simulink model "flightSimulation"  (R2018a)
settings: Solver=FixedStepAuto  StartTime=0  StopTime=end_time  FixedStep=0.005  RelTol=1e-3  EnableMultiTasking=on
values from neighbouring files (symbols this model uses):
  initPosLLA = [37.6287386167 -122.393391133 100]    [cmdh.mat]    (also in cmdyaw.mat)
  mass = 1.53    [cmdh.mat]    (also in cmdyaw.mat)
  Ts = 0.01    [cmdh.mat]    (also in cmdyaw.mat)
undefined symbols (not defined in the file or in its folder): B, Earth, ft, m, p_limits, s, sigbuilder_block, sw_turb, umax, umin, Vehicle, WGS84
libraries: simulink x23, aerolibactuator x15, dspswit3 x12, dspsrcs4 x10, dsparch4 x7, aerolibconvert2 x4, aerolibanimutils x2, qcatlib x2, aerolibfltsims x2, aerolibutil x2, shared6dof x1, aerolibtransform2 x1
(part 3 of 4)

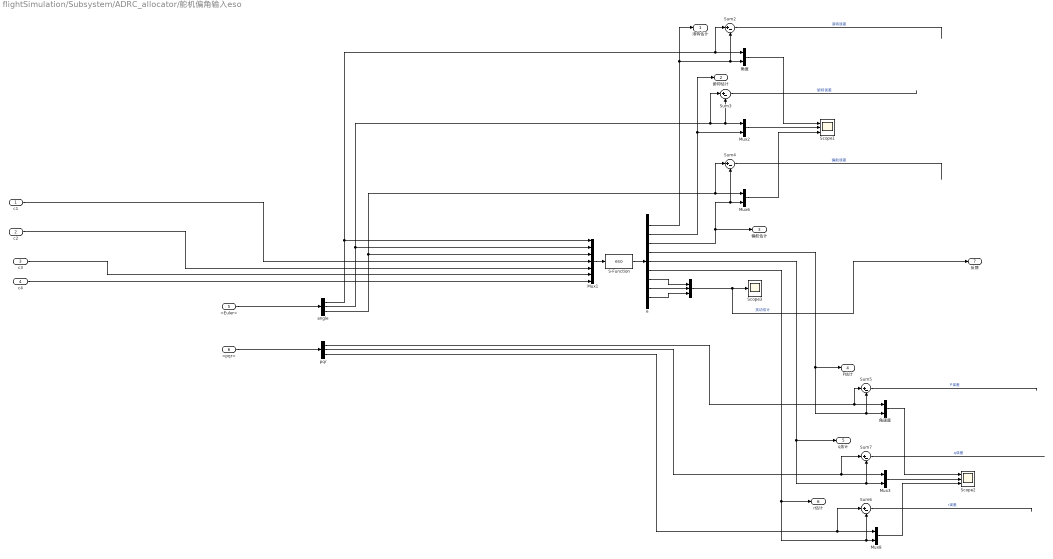
== system flightSimulation/Subsystem/ADRC_allocator/舵机偏角输入eso ==
  c1 : Inport
  c2 : Inport  Port=2
  c3 : Inport  Port=3
  c4 : Inport  Port=4
  <Euler> : Inport  Port=5
  <pqr> : Inport  Port=6
  " " : Mux  Inputs=3
  Mux1 : Mux  Inputs=7
  Mux{2..3,6,8} (4 alike) : Mux  Inputs=2
  S-Function : S-Function  FunctionName=eso  SFunctionDeploymentMode=off  EnableBusSupport=off
  Scope1 : Scope  NumInputPorts=3
  Scope2 : Scope  NumInputPorts=3
  Scope3 : Scope
  Sum{2..7} (6 alike) : Sum  Inputs=|+-
  angle : Demux  Outputs=3
  e : Demux  Outputs=9
  pqr : Demux  Outputs=3
  角度 : Mux  Inputs=2
  角速度 : Mux  Inputs=2
  滚转估计 : Outport
  俯仰估计 : Outport  Port=2
  偏航估计 : Outport  Port=3
  P估计 : Outport  Port=4
  q估计 : Outport  Port=5
  r估计 : Outport  Port=6
  反馈 : Outport  Port=7
  wires:
  e/1 -> 滚转估计/1, Sum2/2, 角度/2
  e/4 -> P估计/1, Sum5/2, 角速度/2
  pqr/1 -> Sum5/1, 角速度/1
  angle/1 -> Sum2/1, 角度/1, Mux1/1
  c3/1 -> Mux1/6
  Sum4/1 -> ?  "偏航误差"
  e/8 -> " "/2
  angle/2 -> Mux2/1, Sum3/2, Sum3/1, Mux1/2
  c2/1 -> Mux1/5
  e/6 -> r估计/1, Mux8/2, Sum6/2
  e/5 -> q估计/1, Sum7/2, Mux3/2
  c4/1 -> Mux1/7
  angle/3 -> Sum4/1, Mux6/1, Mux1/3
  角速度/1 -> Scope2/1
  Mux3/1 -> Scope2/2
  e/3 -> 偏航估计/1, Sum4/2, Mux6/2
  Sum5/1 -> ?  "P误差"
  pqr/3 -> Sum6/1, Mux8/1
  角度/1 -> Scope1/1
  S-Function/1 -> e/1
  pqr/2 -> Sum7/1, Mux3/1
  <Euler>/1 -> angle/1
  Mux6/1 -> Scope1/3
  e/2 -> 俯仰估计/1, Mux2/2
  Mux2/1 -> Scope1/2
  e/7 -> " "/1
  Sum7/1 -> ?  "q误差"
  Mux1/1 -> S-Function/1
  Mux8/1 -> Scope2/3
  e/9 -> " "/3
  Sum6/1 -> ?  "r误差"
  c1/1 -> Mux1/4
  Sum3/1 -> ?  "俯仰误差"
  Sum2/1 -> ?  "滚转误差"
  <pqr>/1 -> pqr/1
  " "/1 -> 反馈/1, Scope3/1  "扰动估计"

== system flightSimulation/Subsystem/ADRC_allocator1/Subsystem ==
  q : Inport
  p : Inport  Port=2
  In3 : Inport  Port=3
  Divide : Product  Inputs=*/
  Gain : Gain  Gain=-1225^2/9.788
  Product : Product
  Saturation1 : Saturate  UpperLimit=1  LowerLimit=0.5
  Sqrt : Sqrt  SaturateOnIntegerOverflow=on
  Trigonometric Function : Trigonometry  Operator=cos
  Trigonometric Function1 : Trigonometry  Operator=cos
  speed : Outport
  wires:
  Saturation1/1 -> Divide/2
  Trigonometric Function/1 -> Product/1
  In3/1 -> Divide/1
  Trigonometric Function1/1 -> Product/2
  p/1 -> Trigonometric Function/1
  Product/1 -> Saturation1/1
  q/1 -> Trigonometric Function1/1
  Divide/1 -> Gain/1
  Gain/1 -> Sqrt/1
  Sqrt/1 -> speed/1

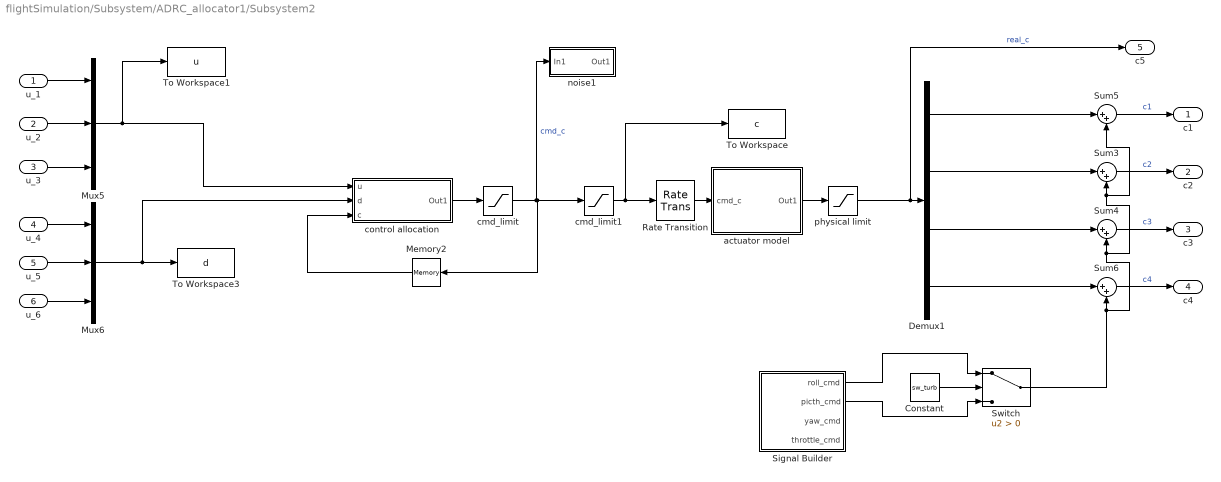
== system flightSimulation/Subsystem/ADRC_allocator1/Subsystem2 ==
  u_1 : Inport
  u_2 : Inport  Port=2
  u_3 : Inport  Port=3
  u_4 : Inport  Port=4
  u_5 : Inport  Port=5
  u_6 : Inport  Port=6
  Constant : Constant  Value=sw_turb
  Demux1 : Demux
  Memory2 : Memory  InitialCondition=[0;0;0;0]  InheritSampleTime=on  LinearizeAsDelay=on
  Mux5 : Mux  Inputs=3
  Mux6 : Mux  Inputs=3
  Rate Transition : RateTransition
  Signal Builder : Subsystem  Tag=STV Subsys  LoadFcn=sigbuilder_block('load');  StartFcn=sigbuilder_block('start');  StopFcn=sigbuilder_block('stop');  ClipboardFcn=sigbuilder_block('clipboard');  mask(Sigbuilder block){tuvar=[0:10]}
      mask help: Simulink:masks:SigbuilderBlock_MD
      mask init:
      | if ~strcmp(get_param(bdroot(gcbh),'SimulationStatus'),'stopped') tuvar = sigbuilder_block('maskInit'); end
      settings: CopyFcn=sigbuilder_block('copy');  DeleteFcn=sigbuilder_block('delete');  ModelCloseFcn=sigbuilder_block('modelClose');  PreSaveFcn=sigbuilder_block('preSave');  PauseFcn=sigbuilder_block('pause');  ContinueFcn=sigbuilder_block('continue');  NameChangeFcn=sigbuilder_block('namechange');  OpenFcn=sigbuilder_block('open',[336 114 630 307.5 ]);  CloseFcn=sigbuilder_block('close');
      mask Display: plot(0, 0, 100, 100,[2, 2, 32, 32, 2], [68, 8, 8, 68, 68],[32, 2], [38, 38], [32, 19, 2],[53, 60, 44], [32, 17, 17, 2],[16, 16, 31, 31]);txt = getActiveGroup(gcbh);text(2, 100, txt,'verticalAlignment', 'top');
  Sum{3..6} (4 alike) : Sum  Inputs=|++
  Switch : Switch  Criteria=u2 > Threshold
  To Workspace : ToWorkspace  VariableName=c  SaveFormat=Timeseries  SampleTime=0.01
  To Workspace1 : ToWorkspace  VariableName=u  SaveFormat=Timeseries  SampleTime=0.01
  To Workspace3 : ToWorkspace  VariableName=d  SaveFormat=Timeseries  SampleTime=0.01
  actuator model : Subsystem
  cmd_limit : Saturate  UpperLimit=umax  LowerLimit=umin
  cmd_limit1 : Saturate  UpperLimit=umax  LowerLimit=umin
  control allocation : Subsystem  Variant=on
  noise1 : Subsystem
  physical limit : Saturate  UpperLimit=umax  LowerLimit=umin
  c1 : Outport
  c2 : Outport  Port=2
  c3 : Outport  Port=3
  c4 : Outport  Port=4
  c5 : Outport  Port=5
  wires:
  u_3/1 -> Mux5/3
  u_1/1 -> Mux5/1
  u_2/1 -> Mux5/2
  u_4/1 -> Mux6/1
  u_5/1 -> Mux6/2
  u_6/1 -> Mux6/3
  Sum5/1 -> c1/1  "c1"
  Sum3/1 -> c2/1  "c2"
  Sum4/1 -> c3/1  "c3"
  Sum6/1 -> c4/1  "c4"
  Memory2/1 -> control allocation/3(c)
  Demux1/1 -> Sum5/1
  Demux1/2 -> Sum3/1
  Demux1/3 -> Sum4/1
  Demux1/4 -> Sum6/1
  Mux6/1 -> control allocation/2(d), To Workspace3/1
  control allocation/1(Out1) -> cmd_limit/1
  Signal Builder/1(roll_cmd) -> Switch/1
  Signal Builder/2(picth_cmd) -> Switch/3
  Constant/1 -> Switch/2
  Switch/1 -> Sum5/2, Sum3/2, Sum4/2, Sum6/2
  Mux5/1 -> To Workspace1/1, control allocation/1(u)
  cmd_limit/1 -> noise1/1(In1), cmd_limit1/1, Memory2/1  "cmd_c"
  physical limit/1 -> c5/1, Demux1/1  "real_c"
  actuator model/1(Out1) -> physical limit/1
  cmd_limit1/1 -> Rate Transition/1, To Workspace/1
  Rate Transition/1 -> actuator model/1(cmd_c)

== system flightSimulation/Subsystem/ADRC_allocator1/input noise ==
  In1 : Inport
  In2 : Inport  Port=2
  In3 : Inport  Port=3
  Colored Noise : dspsrcs4/Colored Noise  Color=white  InverseFrequencyPower=1.55  NumChannels=1  OutputDataType=double  SamplesPerFrame=1  SampleTime=1  RandomStream=mt19937ar with seed  Seed=randperm(100000,1)  SimulateUsing=Interpreted execution
      settings: SourceProductName=DSP System Toolbox  SourceProductBaseCode=DS
  Colored Noise1 : dspsrcs4/Colored Noise  Color=white  InverseFrequencyPower=1.55  NumChannels=1  OutputDataType=double  SamplesPerFrame=1  SampleTime=2  RandomStream=mt19937ar with seed  Seed=randperm(100000,1)  SimulateUsing=Interpreted execution
      settings: SourceProductName=DSP System Toolbox  SourceProductBaseCode=DS
  Colored Noise2 : dspsrcs4/Colored Noise  Color=white  InverseFrequencyPower=1.55  NumChannels=1  OutputDataType=double  SamplesPerFrame=1  SampleTime=0.5  RandomStream=mt19937ar with seed  Seed=randperm(100000,1)  SimulateUsing=Interpreted execution
      settings: SourceProductName=DSP System Toolbox  SourceProductBaseCode=DS
  Gain : Gain  Gain=0.002
  Gain1 : Gain  Gain=0.002
  Gain2 : Gain  Gain=0.003
  Mux1 : Mux  Inputs=2
  Mux2 : Mux  Inputs=2
  Mux3 : Mux  Inputs=2
  Random Number : RandomNumber  Variance=1.8365e-4  Seed=randperm(100000,1)
  Random Number1 : RandomNumber  Variance=1e-4  Seed=randperm(100000,1)
  Random Number2 : RandomNumber  Variance=1.4679e-6  Seed=randperm(100000,1)
  Scope3 : Scope  NumInputPorts=3
  Sum1 : Sum  Inputs=|++
  Sum3 : Sum  Inputs=|++
  Sum4 : Sum  Inputs=|++
  Out1 : Outport
  Out2 : Outport  Port=2
  Out3 : Outport  Port=3
  wires:
  In1/1 -> Mux1/1, Sum1/2
  In2/1 -> Mux2/1, Sum3/2
  In3/1 -> Mux3/1, Sum4/2
  Sum1/1 -> Mux1/2, Out1/1
  Sum4/1 -> Mux3/2, Out3/1
  Mux3/1 -> Scope3/3
  Mux2/1 -> Scope3/2
  Mux1/1 -> Scope3/1
  Colored Noise/1 -> Gain/1
  Colored Noise1/1 -> Gain1/1
  Colored Noise2/1 -> Gain2/1
  Sum3/1 -> Mux2/2, Out2/1

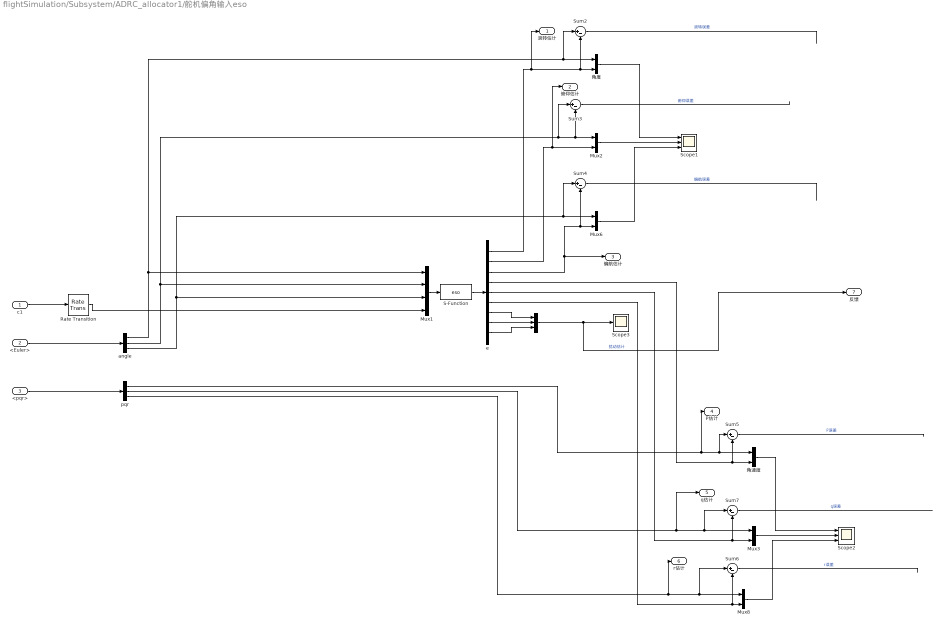
== system flightSimulation/Subsystem/ADRC_allocator1/舵机偏角输入eso ==
  c1 : Inport
  <Euler> : Inport  Port=2
  <pqr> : Inport  Port=3
  " " : Mux  Inputs=3
  Mux1 : Mux
  Mux{2..3,6,8} (4 alike) : Mux  Inputs=2
  Rate Transition : RateTransition  OutPortSampleTime=0.01
  S-Function : S-Function  FunctionName=eso  SFunctionDeploymentMode=off  EnableBusSupport=off
  Scope1 : Scope  NumInputPorts=3
  Scope2 : Scope  NumInputPorts=3
  Scope3 : Scope
  Sum{2..7} (6 alike) : Sum  Inputs=|+-
  angle : Demux  Outputs=3
  e : Demux  Outputs=9
  pqr : Demux  Outputs=3
  角度 : Mux  Inputs=2
  角速度 : Mux  Inputs=2
  滚转估计 : Outport
  俯仰估计 : Outport  Port=2
  偏航估计 : Outport  Port=3
  P估计 : Outport  Port=4
  q估计 : Outport  Port=5
  r估计 : Outport  Port=6
  反馈 : Outport  Port=7
  wires:
  e/1 -> 滚转估计/1, Sum2/2, 角度/2
  e/4 -> Sum5/2, 角速度/2
  pqr/1 -> P估计/1, Sum5/1, 角速度/1
  angle/1 -> Sum2/1, 角度/1, Mux1/1
  Sum4/1 -> ?  "偏航误差"
  e/8 -> " "/2
  angle/2 -> Mux2/1, Sum3/2, Sum3/1, Mux1/2
  e/6 -> Mux8/2, Sum6/2
  e/5 -> Sum7/2, Mux3/2
  angle/3 -> Mux6/1, Sum4/1, Mux1/3
  角速度/1 -> Scope2/1
  Mux3/1 -> Scope2/2
  e/3 -> 偏航估计/1, Sum4/2, Mux6/2
  Sum5/1 -> ?  "P误差"
  pqr/3 -> r估计/1, Sum6/1, Mux8/1
  角度/1 -> Scope1/1
  S-Function/1 -> e/1
  pqr/2 -> q估计/1, Sum7/1, Mux3/1
  <Euler>/1 -> angle/1
  Mux6/1 -> Scope1/3
  e/2 -> 俯仰估计/1, Mux2/2
  Mux2/1 -> Scope1/2
  e/7 -> " "/1
  Sum7/1 -> ?  "q误差"
  Mux1/1 -> S-Function/1
  Mux8/1 -> Scope2/3
  e/9 -> " "/3
  Sum6/1 -> ?  "r误差"
  c1/1 -> Rate Transition/1
  Sum3/1 -> ?  "俯仰误差"
  Sum2/1 -> ?  "滚转误差"
  <pqr>/1 -> pqr/1
  " "/1 -> 反馈/1, Scope3/1  "扰动估计"
  Rate Transition/1 -> Mux1/4

== system flightSimulation/Subsystem/PID/Signal Builder ==
  Demux : Demux  Tag=STV Demux
  FromWs : FromWorkspace  Tag=STV FromWs  VariableName=tuvar  SampleTime=0
      SigBuilderData=|
      | common.afterFinalStr = 'Extrapolate'
      | common.sampleTime = 0
      | dataSet.timeRange = [0 50]
      | dataSet.name = 'Group 1'
      | sbobj.Groups.Name = 'Group 1'
      | sbobj.Groups.Signals(1).Name = 'roll_cmd'
      | sbobj.Groups.Signals(1).XData = [0 6 6 8.55 8.55 10.7 10.7 13 13 50]
      | sbobj.Groups.Signals(1).YData = [0 0 0.05 0.05 0 0 -0.05 -0.05 0 0]
      | sbobj.Groups.Signals(2).Name = 'picth_cmd'
      | sbobj.Groups.Signals(2).XData = [0 14.9 14.9 17.5 17.5 20.8 50]
      | sbobj.Groups.Signals(2).YData = [0 0 0.05 0.05 0 0 0]
      | sbobj.Groups.Signals(3).Name = 'yaw_cmd'
      | sbobj.Groups.Signals(3).XData = [0 33.4 33.4 39.4 39.4 40.9 40.9 46.65 46.65 50]
      | sbobj.Groups.Signals(3).YData = [0 0 0.1 0.1 0 0 -0.1 -0.1 0 0]
      | sbobj.Groups.Signals(4).Name = 'throttle_cmd'
      | sbobj.Groups.Signals(4).XData = [0 10 21.35 21.35 26.15 32.4 50]
      | sbobj.Groups.Signals(4).YData = [0 -1.8 -1.8 -3.8 -3.8 -3.8 -3.8]
      | sbobj.Groups.TimeRange = [0 50]
  roll_cmd : Outport  Tag=STV Outport
  picth_cmd : Outport  Tag=STV Outport  Port=2
  yaw_cmd : Outport  Tag=STV Outport  Port=3
  throttle_cmd : Outport  Tag=STV Outport  Port=4
  wires:
  Demux/1 -> roll_cmd/1
  FromWs/1 -> Demux/1
  Demux/2 -> picth_cmd/1
  Demux/3 -> yaw_cmd/1
  Demux/4 -> throttle_cmd/1

== system flightSimulation/Subsystem/PID/Subsystem ==
  In1 : Inport
  In2 : Inport  Port=2
  In3 : Inport  Port=3
  Divide : Product  Inputs=*/
  Gain : Gain  Gain=-1225^2/9.788
  Product : Product
  Saturation1 : Saturate  UpperLimit=1  LowerLimit=0.5
  Sqrt : Sqrt  SaturateOnIntegerOverflow=on
  Trigonometric Function : Trigonometry  Operator=cos
  Trigonometric Function1 : Trigonometry  Operator=cos
  speed : Outport
  wires:
  Saturation1/1 -> Divide/2
  Trigonometric Function/1 -> Product/1
  In3/1 -> Divide/1
  Trigonometric Function1/1 -> Product/2
  In2/1 -> Trigonometric Function/1
  Product/1 -> Saturation1/1
  In1/1 -> Trigonometric Function1/1
  Divide/1 -> Gain/1
  Gain/1 -> Sqrt/1
  Sqrt/1 -> speed/1

== system flightSimulation/Subsystem/PID/gyro ==
  u_p : Inport
  p : Inport  Port=2
  u_q : Inport  Port=3
  q : Inport  Port=4
  u_r : Inport  Port=5
  speed : Inport  Port=6
  Add1 : Sum
  Add2 : Sum  Inputs=+-
  Add3 : Sum  Inputs=+-
  Constant1 : Constant  Value=0.000029
  Constant2 : Constant  Value=0.04238
  Product{,1..3} (4 alike) : Product
  u_1 : Outport
  u_2 : Outport  Port=2
  u_3 : Outport  Port=3
  wires:
  Add3/1 -> u_3/1
  Add1/1 -> u_1/1
  Constant1/1 -> Product1/1, Product/2
  q/1 -> Product/1
  Product1/1 -> Product2/1
  Constant2/1 -> Add3/2
  u_p/1 -> Add1/2
  p/1 -> Product1/2
  Add2/1 -> u_2/1
  Product3/1 -> Add1/1
  speed/1 -> Product3/2, Product2/2
  Product/1 -> Product3/1
  Product2/1 -> Add2/2
  u_q/1 -> Add2/1
  u_r/1 -> Add3/1

== system flightSimulation/Subsystem/PID/舵面分配 ==
  u_1 : Inport
  u_2 : Inport  Port=2
  u_3 : Inport  Port=3
  Constant1 : Constant  Value=0.3
  Demux3 : Demux
  Gain{,1..3} (4 alike) : Gain
  Linear Second-Order Actuator3 : aerolibactuator/Linear Second-Order Actuator  wn_fin=100  z_fin=1  fin_act_0=0  fin_act_vel=0
      settings: SourceProductName=Aerospace Blockset  SourceProductBaseCode=AE
  Mux : Mux  Inputs=3
  N-Sample Switch1 : dspswit3/N-Sample Switch  N=1990  reset=off  TriggerType=Rising edge  Ts=0.01
      settings: SourceProductName=DSP System Toolbox  SourceProductBaseCode=DS
  N-Sample Switch2 : dspswit3/N-Sample Switch  N=2000  reset=off  TriggerType=Rising edge  Ts=0.01
      settings: SourceProductName=DSP System Toolbox  SourceProductBaseCode=DS
  Nonlinear Second-Order Actuator{1..4} (4 alike) : aerolibactuator/Nonlinear Second-Order Actuator  wn_fin=100  z_fin=1  fin_max=60*pi/180  fin_min=-60*pi/180  fin_maxrate=380*pi/180  fin_act_0=0  fin_act_vel=0
      settings: SourceProductName=Aerospace Blockset  SourceProductBaseCode=AE
  Nonlinear Second-Order Actuator6 : aerolibactuator/Nonlinear Second-Order Actuator  wn_fin=100  z_fin=1  fin_max=60*pi/180  fin_min=-60*pi/180  fin_maxrate=500*pi/180  fin_act_0=0  fin_act_vel=0
      settings: SourceProductName=Aerospace Blockset  SourceProductBaseCode=AE
  Saturation{1..4} (4 alike) : Saturate  UpperLimit=0.3491  LowerLimit=-0.3491
  Sum1 : Sum  Inputs=|++
  Sum2 : Sum  Inputs=|+-
  Sum3 : Sum  Inputs=|+-
  Transfer Fcn : TransferFcn  Denominator=[0.0001144 0.02139 1]
  Transfer Fcnnon3 : TransferFcn  Denominator=[0.01^2 2*0.01*0.999 1]
  inv : MATLAB Function  TreatAsAtomicUnit=on
  c1 : Outport
  c2 : Outport  Port=2
  c3 : Outport  Port=3
  c4 : Outport  Port=4
  wires:
  inv/1(y) -> Demux3/1
  u_3/1 -> Mux/3
  u_2/1 -> Mux/2
  u_1/1 -> Mux/1
  Demux3/2 -> Saturation2/1
  Demux3/3 -> Sum2/1
  Demux3/4 -> Saturation4/1
  Transfer Fcn/1 -> ?
  Mux/1 -> inv/1(u)
  Gain1/1 -> c2/1  "c2"
  Gain3/1 -> c4/1  "c4"
  Nonlinear Second-Order Actuator3/1 -> Gain3/1
  Transfer Fcnnon3/1 -> Sum3/1
  Nonlinear Second-Order Actuator2/1 -> Gain2/1
  Nonlinear Second-Order Actuator1/1 -> Gain1/1
  Gain/1 -> c1/1  "c1"
  Gain2/1 -> c3/1  "c3"
  Saturation1/1 -> Transfer Fcnnon3/1, Nonlinear Second-Order Actuator4/1
  Saturation3/1 -> Nonlinear Second-Order Actuator2/1
  Saturation4/1 -> Nonlinear Second-Order Actuator3/1
  Saturation2/1 -> Nonlinear Second-Order Actuator1/1
  Nonlinear Second-Order Actuator4/1 -> Gain/1, Sum3/2
  Demux3/1 -> Sum1/1
  Sum1/1 -> Saturation1/1
  Sum2/1 -> Saturation3/1
  N-Sample Switch1/1 -> N-Sample Switch2/1
  Constant1/1 -> N-Sample Switch1/2

== system flightSimulation/Subsystem/PID_allocator/Subsystem ==
  In1 : Inport
  In2 : Inport  Port=2
  In3 : Inport  Port=3
  Divide : Product  Inputs=*/
  Gain : Gain  Gain=-1225^2/9.788
  Product : Product
  Saturation1 : Saturate  UpperLimit=1  LowerLimit=0.5
  Sqrt : Sqrt  SaturateOnIntegerOverflow=on
  Trigonometric Function : Trigonometry  Operator=cos
  Trigonometric Function1 : Trigonometry  Operator=cos
  speed : Outport
  wires:
  Saturation1/1 -> Divide/2
  Trigonometric Function/1 -> Product/1
  In3/1 -> Divide/1
  Trigonometric Function1/1 -> Product/2
  In2/1 -> Trigonometric Function/1
  Product/1 -> Saturation1/1
  In1/1 -> Trigonometric Function1/1
  Divide/1 -> Gain/1
  Gain/1 -> Sqrt/1
  Sqrt/1 -> speed/1

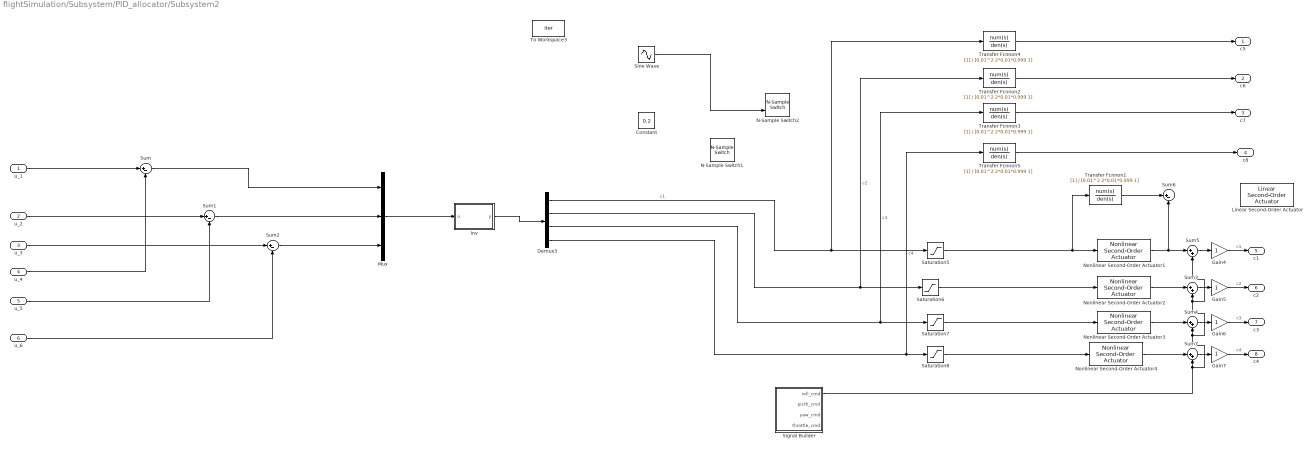
== system flightSimulation/Subsystem/PID_allocator/Subsystem2 ==
  u_1 : Inport
  u_2 : Inport  Port=2
  u_3 : Inport  Port=3
  u_4 : Inport  Port=4
  u_5 : Inport  Port=5
  u_6 : Inport  Port=6
  Constant : Constant  Value=0.2
  Demux3 : Demux
  Gain{4..7} (4 alike) : Gain
  Linear Second-Order Actuator : aerolibactuator/Linear Second-Order Actuator  wn_fin=100  z_fin=1  fin_act_0=0  fin_act_vel=0
      settings: SourceProductName=Aerospace Blockset  SourceProductBaseCode=AE
  Mux : Mux  Inputs=3
  N-Sample Switch1 : dspswit3/N-Sample Switch  N=2000  reset=off  TriggerType=Rising edge  Ts=0.01
      settings: SourceProductName=DSP System Toolbox  SourceProductBaseCode=DS
  N-Sample Switch2 : dspswit3/N-Sample Switch  N=3000  reset=off  TriggerType=Rising edge  Ts=0.01
      settings: SourceProductName=DSP System Toolbox  SourceProductBaseCode=DS
  Nonlinear Second-Order Actuator{1..4} (4 alike) : aerolibactuator/Nonlinear Second-Order Actuator  wn_fin=100  z_fin=1  fin_max=60*pi/180  fin_min=-60*pi/180  fin_maxrate=380*pi/180  fin_act_0=0  fin_act_vel=0
      settings: SourceProductName=Aerospace Blockset  SourceProductBaseCode=AE
  Saturation{5..8} (4 alike) : Saturate  UpperLimit=15*pi/180  LowerLimit=-15*pi/180
  Signal Builder : Subsystem  Tag=STV Subsys  LoadFcn=sigbuilder_block('load');  StartFcn=sigbuilder_block('start');  StopFcn=sigbuilder_block('stop');  ClipboardFcn=sigbuilder_block('clipboard');  mask(Sigbuilder block){tuvar=[0:10]}
      mask help: Simulink:masks:SigbuilderBlock_MD
      mask init:
      | if ~strcmp(get_param(bdroot(gcbh),'SimulationStatus'),'stopped') tuvar = sigbuilder_block('maskInit'); end
      settings: CopyFcn=sigbuilder_block('copy');  DeleteFcn=sigbuilder_block('delete');  ModelCloseFcn=sigbuilder_block('modelClose');  PreSaveFcn=sigbuilder_block('preSave');  PauseFcn=sigbuilder_block('pause');  ContinueFcn=sigbuilder_block('continue');  NameChangeFcn=sigbuilder_block('namechange');  OpenFcn=sigbuilder_block('open',[108 142.5 949.5 468.75 ]);  CloseFcn=sigbuilder_block('close');
      mask Display: plot(0, 0, 100, 100,[2, 2, 32, 32, 2], [68, 8, 8, 68, 68],[32, 2], [38, 38], [32, 19, 2],[53, 60, 44], [32, 17, 17, 2],[16, 16, 31, 31]);txt = getActiveGroup(gcbh);text(2, 100, txt,'verticalAlignment', 'top');
  Sine Wave : Sin  Amplitude=0.2  Frequency=2*pi/2.5  SampleTime=0.01
  Sum{,1..2,6} (4 alike) : Sum  Inputs=|+-
  Sum{3..5,7} (4 alike) : Sum  Inputs=|++
  To Workspace3 : ToWorkspace  VariableName=iter  SaveFormat=Timeseries  SampleTime=-1
  Transfer Fcnnon{1..5} (5 alike) : TransferFcn  Denominator=[0.01^2 2*0.01*0.999 1]
  inv : MATLAB Function  TreatAsAtomicUnit=on
  c5 : Outport
  c6 : Outport  Port=2
  c7 : Outport  Port=3
  c8 : Outport  Port=4
  c1 : Outport  Port=5
  c2 : Outport  Port=6
  c3 : Outport  Port=7
  c4 : Outport  Port=8
  wires:
  u_3/1 -> Sum2/1
  u_1/1 -> Sum/1
  u_2/1 -> Sum1/1
  Sum2/1 -> Mux/3
  Sum/1 -> Mux/1
  Sum1/1 -> Mux/2
  Transfer Fcnnon1/1 -> Sum6/1
  Gain7/1 -> c4/1  "c4"
  Gain6/1 -> c3/1  "c3"
  Gain4/1 -> c1/1  "c1"
  Gain5/1 -> c2/1  "c2"
  Demux3/1 -> Saturation5/1, Transfer Fcnnon4/1  "c1"
  Demux3/4 -> Saturation8/1, Transfer Fcnnon5/1  "c4"
  Demux3/3 -> Transfer Fcnnon3/1, Saturation7/1  "c3"
  Demux3/2 -> Saturation6/1, Transfer Fcnnon2/1  "c2"
  Transfer Fcnnon4/1 -> c5/1
  Transfer Fcnnon2/1 -> c6/1
  Transfer Fcnnon3/1 -> c7/1
  Transfer Fcnnon5/1 -> c8/1
  Saturation5/1 -> Nonlinear Second-Order Actuator1/1, Transfer Fcnnon1/1
  Saturation6/1 -> Nonlinear Second-Order Actuator2/1
  Saturation7/1 -> Nonlinear Second-Order Actuator3/1
  Saturation8/1 -> Nonlinear Second-Order Actuator4/1
  Sine Wave/1 -> N-Sample Switch2/2
  Nonlinear Second-Order Actuator1/1 -> Sum5/1, Sum6/2
  Nonlinear Second-Order Actuator2/1 -> Sum3/1
  Nonlinear Second-Order Actuator3/1 -> Sum4/1
  Nonlinear Second-Order Actuator4/1 -> Sum7/1
  Mux/1 -> inv/1(u)
  u_4/1 -> Sum/2
  u_5/1 -> Sum1/2
  u_6/1 -> Sum2/2
  Sum5/1 -> Gain4/1
  Sum3/1 -> Gain5/1
  Sum4/1 -> Gain6/1
  Sum7/1 -> Gain7/1
  Signal Builder/1(roll_cmd) -> Sum5/2, Sum3/2, Sum4/2, Sum7/2
  inv/1(y) -> Demux3/1

== system flightSimulation/Subsystem/PID_allocator/gyro ==
  u_p : Inport
  p : Inport  Port=2
  u_q : Inport  Port=3
  q : Inport  Port=4
  u_r : Inport  Port=5
  speed : Inport  Port=6
  Add1 : Sum
  Add2 : Sum  Inputs=+-
  Add3 : Sum  Inputs=+-
  Constant1 : Constant  Value=0.000029
  Constant2 : Constant  Value=0.04238
  Product{,1..3} (4 alike) : Product
  u_1 : Outport
  u_2 : Outport  Port=2
  u_3 : Outport  Port=3
  wires:
  Add3/1 -> u_3/1
  Add1/1 -> u_1/1
  Constant1/1 -> Product1/1, Product/2
  q/1 -> Product/1
  Product1/1 -> Product2/1
  Constant2/1 -> Add3/2
  u_p/1 -> Add1/2
  p/1 -> Product1/2
  Add2/1 -> u_2/1
  Product3/1 -> Add1/1
  speed/1 -> Product3/2, Product2/2
  Product/1 -> Product3/1
  Product2/1 -> Add2/2
  u_q/1 -> Add2/1
  u_r/1 -> Add3/1

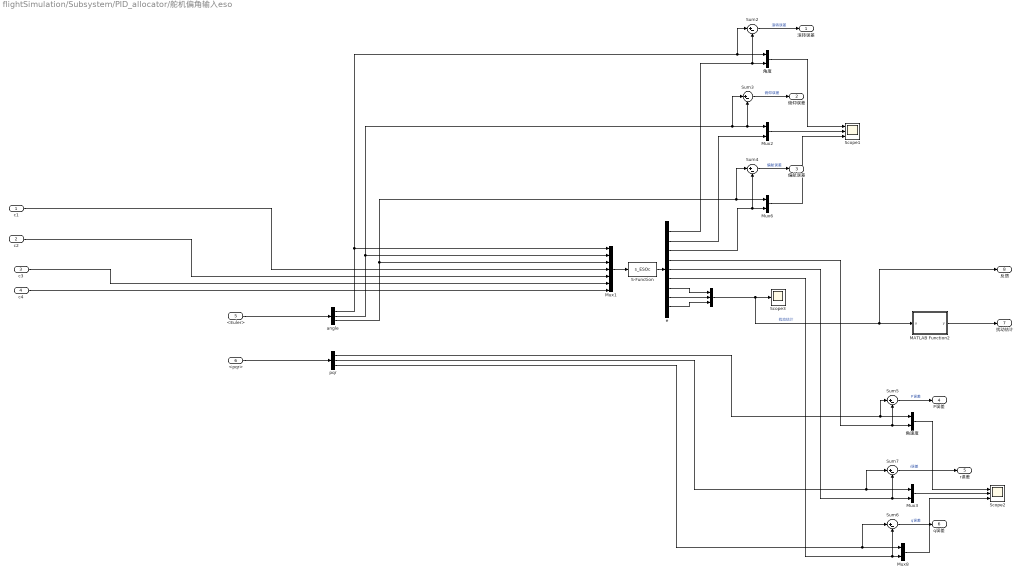
== system flightSimulation/Subsystem/PID_allocator/舵机偏角输入eso ==
  c1 : Inport
  c2 : Inport  Port=2
  c3 : Inport  Port=3
  c4 : Inport  Port=4
  <Euler> : Inport  Port=5
  <pqr> : Inport  Port=6
  " " : Mux  Inputs=3
  MATLAB Function2 : MATLAB Function  TreatAsAtomicUnit=on
  Mux1 : Mux  Inputs=7
  Mux{2..3,6,8} (4 alike) : Mux  Inputs=2
  S-Function : S-Function  FunctionName=s_ESOc  SFunctionDeploymentMode=off  EnableBusSupport=off
  Scope1 : Scope  NumInputPorts=3
  Scope2 : Scope  NumInputPorts=3
  Scope3 : Scope
  Sum{2..7} (6 alike) : Sum  Inputs=|+-
  angle : Demux  Outputs=3
  e : Demux  Outputs=9
  pqr : Demux  Outputs=3
  角度 : Mux  Inputs=2
  角速度 : Mux  Inputs=2
  滚转误差 : Outport
  俯仰误差 : Outport  Port=2
  偏航误差 : Outport  Port=3
  P误差 : Outport  Port=4
  r误差 : Outport  Port=5
  q误差 : Outport  Port=6
  扰动估计 : Outport  Port=7
  反馈 : Outport  Port=8
  wires:
  e/1 -> Sum2/2, 角度/2
  e/4 -> Sum5/2, 角速度/2
  pqr/1 -> Sum5/1, 角速度/1
  angle/1 -> Sum2/1, 角度/1, Mux1/1
  c3/1 -> Mux1/6
  Sum4/1 -> 偏航误差/1  "偏航误差"
  e/8 -> " "/2
  angle/2 -> Mux2/1, Sum3/2, Sum3/1, Mux1/2
  c2/1 -> Mux1/5
  e/6 -> Mux8/2, Sum6/2
  e/5 -> Sum7/2, Mux3/2
  c4/1 -> Mux1/7
  angle/3 -> Sum4/1, Mux6/1, Mux1/3
  角速度/1 -> Scope2/1
  Mux3/1 -> Scope2/2
  e/3 -> Sum4/2, Mux6/2
  Sum5/1 -> P误差/1  "P误差"
  pqr/3 -> Sum6/1, Mux8/1
  角度/1 -> Scope1/1
  S-Function/1 -> e/1
  pqr/2 -> Sum7/1, Mux3/1
  <Euler>/1 -> angle/1
  Mux6/1 -> Scope1/3
  e/2 -> Mux2/2
  Mux2/1 -> Scope1/2
  e/7 -> " "/1
  Sum7/1 -> r误差/1  "r误差"
  Mux1/1 -> S-Function/1
  Mux8/1 -> Scope2/3
  e/9 -> " "/3
  Sum6/1 -> q误差/1  "q误差"
  c1/1 -> Mux1/4
  Sum3/1 -> 俯仰误差/1  "俯仰误差"
  Sum2/1 -> 滚转误差/1  "滚转误差"
  <pqr>/1 -> pqr/1
  " "/1 -> MATLAB Function2/1(u), 反馈/1, Scope3/1  "扰动估计"
  MATLAB Function2/1(y) -> 扰动估计/1

== system flightSimulation/Subsystem/PID_allocator1/Subsystem ==
  In1 : Inport
  In2 : Inport  Port=2
  In3 : Inport  Port=3
  Divide : Product  Inputs=*/
  Gain : Gain  Gain=-1225^2/9.788
  Product : Product
  Saturation1 : Saturate  UpperLimit=1  LowerLimit=0.5
  Sqrt : Sqrt  SaturateOnIntegerOverflow=on
  Trigonometric Function : Trigonometry  Operator=cos
  Trigonometric Function1 : Trigonometry  Operator=cos
  speed : Outport
  wires:
  Saturation1/1 -> Divide/2
  Trigonometric Function/1 -> Product/1
  In3/1 -> Divide/1
  Trigonometric Function1/1 -> Product/2
  In2/1 -> Trigonometric Function/1
  Product/1 -> Saturation1/1
  In1/1 -> Trigonometric Function1/1
  Divide/1 -> Gain/1
  Gain/1 -> Sqrt/1
  Sqrt/1 -> speed/1

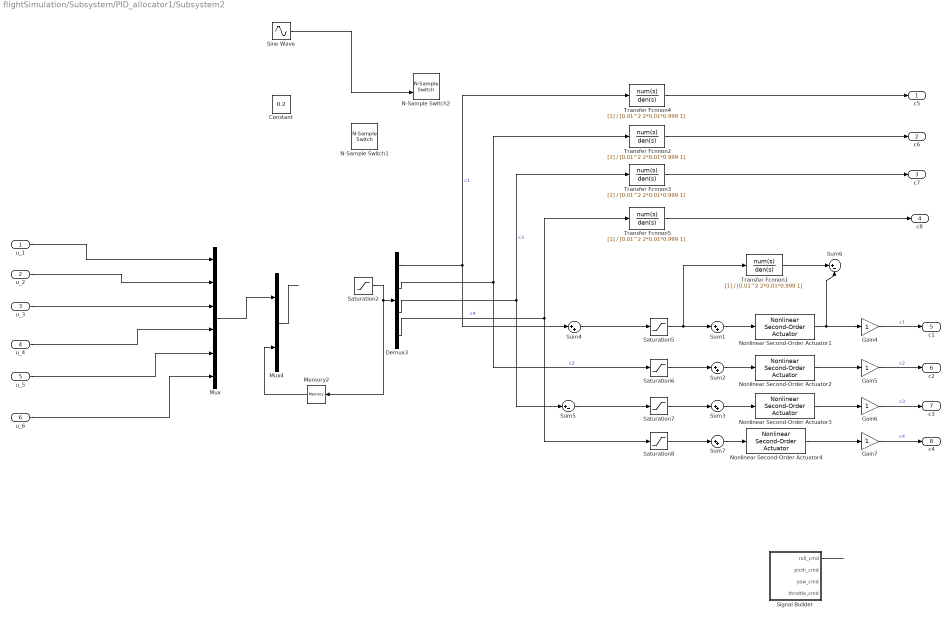
== system flightSimulation/Subsystem/PID_allocator1/Subsystem2 ==
  u_1 : Inport
  u_2 : Inport  Port=2
  u_3 : Inport  Port=3
  u_4 : Inport  Port=4
  u_5 : Inport  Port=5
  u_6 : Inport  Port=6
  Constant : Constant  Value=0.2
  Demux3 : Demux
  Gain{4..7} (4 alike) : Gain
  Memory2 : Memory  InitialCondition=[0;0;0;0]  InheritSampleTime=on  LinearizeAsDelay=on
  Mux : Mux  Inputs=6
  Mux4 : Mux  Inputs=2
  N-Sample Switch1 : dspswit3/N-Sample Switch  N=2000  reset=off  TriggerType=Rising edge  Ts=0.01
      settings: SourceProductName=DSP System Toolbox  SourceProductBaseCode=DS
  N-Sample Switch2 : dspswit3/N-Sample Switch  N=3000  reset=off  TriggerType=Rising edge  Ts=0.01
      settings: SourceProductName=DSP System Toolbox  SourceProductBaseCode=DS
  Nonlinear Second-Order Actuator{1..4} (4 alike) : aerolibactuator/Nonlinear Second-Order Actuator  wn_fin=100  z_fin=1  fin_max=60*pi/180  fin_min=-60*pi/180  fin_maxrate=380*pi/180  fin_act_0=0  fin_act_vel=0
      settings: SourceProductName=Aerospace Blockset  SourceProductBaseCode=AE
  Saturation2 : Saturate  UpperLimit=[p_limits*pi/180;p_limits*pi/180;p_limits*pi/180;p_limits*pi/180]  LowerLimit=-[p_limits*pi/180;p_limits*pi/180;p_limits*pi/180;p_limits*pi/180]
  Saturation{5..8} (4 alike) : Saturate  UpperLimit=20*pi/180  LowerLimit=-20*pi/180
  Signal Builder : Subsystem  Tag=STV Subsys  LoadFcn=sigbuilder_block('load');  StartFcn=sigbuilder_block('start');  StopFcn=sigbuilder_block('stop');  ClipboardFcn=sigbuilder_block('clipboard');  mask(Sigbuilder block){tuvar=[0:10]}
      mask help: Simulink:masks:SigbuilderBlock_MD
      mask init:
      | if ~strcmp(get_param(bdroot(gcbh),'SimulationStatus'),'stopped') tuvar = sigbuilder_block('maskInit'); end
      settings: CopyFcn=sigbuilder_block('copy');  DeleteFcn=sigbuilder_block('delete');  ModelCloseFcn=sigbuilder_block('modelClose');  PreSaveFcn=sigbuilder_block('preSave');  PauseFcn=sigbuilder_block('pause');  ContinueFcn=sigbuilder_block('continue');  NameChangeFcn=sigbuilder_block('namechange');  OpenFcn=sigbuilder_block('open',[108 142.5 949.5 468.75 ]);  CloseFcn=sigbuilder_block('close');
      mask Display: plot(0, 0, 100, 100,[2, 2, 32, 32, 2], [68, 8, 8, 68, 68],[32, 2], [38, 38], [32, 19, 2],[53, 60, 44], [32, 17, 17, 2],[16, 16, 31, 31]);txt = getActiveGroup(gcbh);text(2, 100, txt,'verticalAlignment', 'top');
  Sine Wave : Sin  Amplitude=0.2  Frequency=2*pi/2.5  SampleTime=0.01
  Sum{1..4,7} (5 alike) : Sum  Inputs=|++
  Sum5 : Sum  Inputs=|+-
  Sum6 : Sum  Inputs=|+-
  Transfer Fcnnon{1..5} (5 alike) : TransferFcn  Denominator=[0.01^2 2*0.01*0.999 1]
  c5 : Outport
  c6 : Outport  Port=2
  c7 : Outport  Port=3
  c8 : Outport  Port=4
  c1 : Outport  Port=5
  c2 : Outport  Port=6
  c3 : Outport  Port=7
  c4 : Outport  Port=8
  wires:
  u_3/1 -> Mux/3
  u_1/1 -> Mux/1
  u_2/1 -> Mux/2
  Sum5/1 -> Saturation7/1
  Transfer Fcnnon1/1 -> Sum6/1
  Gain6/1 -> c3/1  "c3"
  Gain4/1 -> c1/1  "c1"
  Gain5/1 -> c2/1  "c2"
  Sum4/1 -> Saturation5/1
  Demux3/1 -> Sum4/1, Transfer Fcnnon4/1  "c1"
  Demux3/4 -> Saturation8/1, Transfer Fcnnon5/1  "c4"
  Demux3/3 -> Sum5/1, Transfer Fcnnon3/1  "c3"
  Demux3/2 -> Saturation6/1, Transfer Fcnnon2/1  "c2"
  Transfer Fcnnon4/1 -> c5/1
  Transfer Fcnnon2/1 -> c6/1
  Transfer Fcnnon3/1 -> c7/1
  Transfer Fcnnon5/1 -> c8/1
  ? -> N-Sample Switch1/1
  Saturation5/1 -> Sum1/1, Transfer Fcnnon1/1
  Saturation6/1 -> Sum2/1
  Saturation7/1 -> Sum3/1
  Saturation8/1 -> Sum7/1
  Sine Wave/1 -> N-Sample Switch2/2
  u_4/1 -> Mux/4
  u_5/1 -> Mux/5
  u_6/1 -> Mux/6
  ? -> Saturation2/1
  Gain7/1 -> c4/1  "c4"
  Nonlinear Second-Order Actuator1/1 -> Gain4/1, Sum6/2
  Nonlinear Second-Order Actuator4/1 -> Gain7/1
  Nonlinear Second-Order Actuator3/1 -> Gain6/1
  Nonlinear Second-Order Actuator2/1 -> Gain5/1
  Sum1/1 -> Nonlinear Second-Order Actuator1/1
  Sum2/1 -> Nonlinear Second-Order Actuator2/1
  Sum3/1 -> Nonlinear Second-Order Actuator3/1
  Sum7/1 -> Nonlinear Second-Order Actuator4/1
  Signal Builder/1(roll_cmd) -> ?
  Mux/1 -> Mux4/1
  Mux4/1 -> ?
  Memory2/1 -> Mux4/2
  Saturation2/1 -> Memory2/1, Demux3/1

== system flightSimulation/Subsystem/PID_allocator1/gyro ==
  u_p : Inport
  p : Inport  Port=2
  u_q : Inport  Port=3
  q : Inport  Port=4
  u_r : Inport  Port=5
  speed : Inport  Port=6
  Add1 : Sum
  Add2 : Sum  Inputs=+-
  Add3 : Sum  Inputs=+-
  Constant1 : Constant  Value=0.000029
  Constant2 : Constant  Value=0.04238
  Product{,1..3} (4 alike) : Product
  u_1 : Outport
  u_2 : Outport  Port=2
  u_3 : Outport  Port=3
  wires:
  Add3/1 -> u_3/1
  Add1/1 -> u_1/1
  Constant1/1 -> Product1/1, Product/2
  q/1 -> Product/1
  Product1/1 -> Product2/1
  Constant2/1 -> Add3/2
  u_p/1 -> Add1/2
  p/1 -> Product1/2
  Add2/1 -> u_2/1
  Product3/1 -> Add1/1
  speed/1 -> Product3/2, Product2/2
  Product/1 -> Product3/1
  Product2/1 -> Add2/2
  u_q/1 -> Add2/1
  u_r/1 -> Add3/1

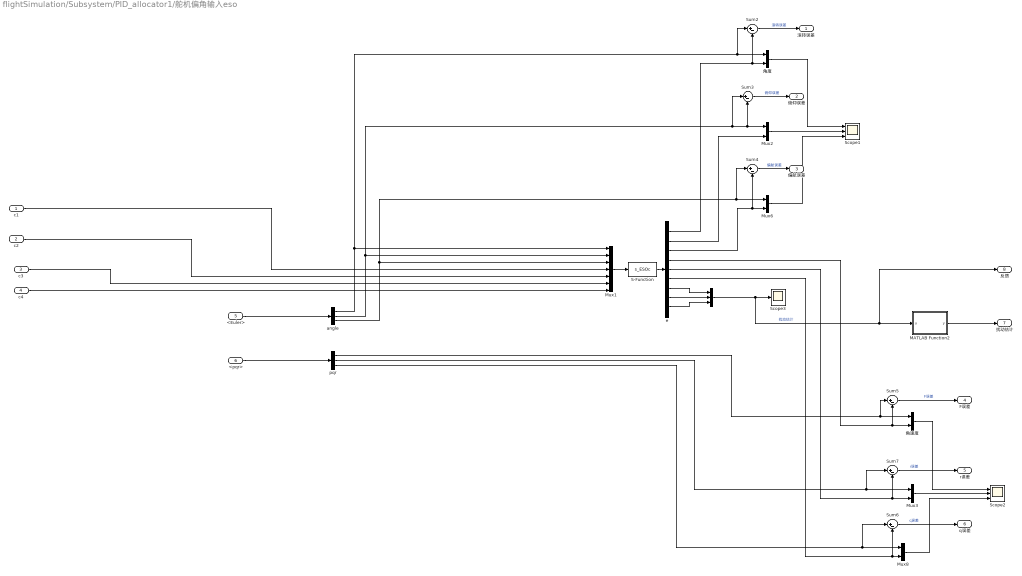
== system flightSimulation/Subsystem/PID_allocator1/舵机偏角输入eso ==
  c1 : Inport
  c2 : Inport  Port=2
  c3 : Inport  Port=3
  c4 : Inport  Port=4
  <Euler> : Inport  Port=5
  <pqr> : Inport  Port=6
  " " : Mux  Inputs=3
  MATLAB Function2 : MATLAB Function  TreatAsAtomicUnit=on
  Mux1 : Mux  Inputs=7
  Mux{2..3,6,8} (4 alike) : Mux  Inputs=2
  S-Function : S-Function  FunctionName=s_ESOc  SFunctionDeploymentMode=off  EnableBusSupport=off
  Scope1 : Scope  NumInputPorts=3
  Scope2 : Scope  NumInputPorts=3
  Scope3 : Scope
  Sum{2..7} (6 alike) : Sum  Inputs=|+-
  angle : Demux  Outputs=3
  e : Demux  Outputs=9
  pqr : Demux  Outputs=3
  角度 : Mux  Inputs=2
  角速度 : Mux  Inputs=2
  滚转误差 : Outport
  俯仰误差 : Outport  Port=2
  偏航误差 : Outport  Port=3
  P误差 : Outport  Port=4
  r误差 : Outport  Port=5
  q误差 : Outport  Port=6
  扰动估计 : Outport  Port=7
  反馈 : Outport  Port=8
  wires:
  e/1 -> Sum2/2, 角度/2
  e/4 -> Sum5/2, 角速度/2
  pqr/1 -> Sum5/1, 角速度/1
  angle/1 -> Sum2/1, 角度/1, Mux1/1
  c3/1 -> Mux1/6
  Sum4/1 -> 偏航误差/1  "偏航误差"
  e/8 -> " "/2
  angle/2 -> Mux2/1, Sum3/2, Sum3/1, Mux1/2
  c2/1 -> Mux1/5
  e/6 -> Mux8/2, Sum6/2
  e/5 -> Sum7/2, Mux3/2
  c4/1 -> Mux1/7
  angle/3 -> Sum4/1, Mux6/1, Mux1/3
  角速度/1 -> Scope2/1
  Mux3/1 -> Scope2/2
  e/3 -> Sum4/2, Mux6/2
  Sum5/1 -> P误差/1  "P误差"
  pqr/3 -> Sum6/1, Mux8/1
  角度/1 -> Scope1/1
  S-Function/1 -> e/1
  pqr/2 -> Sum7/1, Mux3/1
  <Euler>/1 -> angle/1
  Mux6/1 -> Scope1/3
  e/2 -> Mux2/2
  Mux2/1 -> Scope1/2
  e/7 -> " "/1
  Sum7/1 -> r误差/1  "r误差"
  Mux1/1 -> S-Function/1
  Mux8/1 -> Scope2/3
  e/9 -> " "/3
  Sum6/1 -> q误差/1  "q误差"
  c1/1 -> Mux1/4
  Sum3/1 -> 俯仰误差/1  "俯仰误差"
  Sum2/1 -> 滚转误差/1  "滚转误差"
  <pqr>/1 -> pqr/1
  " "/1 -> MATLAB Function2/1(u), 反馈/1, Scope3/1  "扰动估计"
  MATLAB Function2/1(y) -> 扰动估计/1

== system flightSimulation/Visualization/Visualization/FlightGear ==
  Commands : Inport
  States : Inport  Port=2
  Bus Selector : BusSelector  OutputSignals=LLA,Euler
  FlightGear Preconfigured 6DoF Animation : aerolibfltsims/FlightGear Preconfigured 6DoF Animation  xFlightGearVersion=v2017.3  DestinationIpAddress=Visualization.FlightGear.SixDOF.IPAddress  DestinationPort=Visualization.FlightGear.SixDOF.destinationPort  SampleTime=Ts
      settings: SourceProductName=Aerospace Blockset
  Generate Run Script : aerolibfltsims/Generate Run Script  Architecture=Default  dataFlow=Send  GeometryModelName=Model  AirportId=KSFO  RunwayId=10L  InitialAltitude=Visualization.FlightGear.generateRunScript.initialAltitude  InitialHeading=Visualization.FlightGear.generateRunScript.initialHeading  OffsetDistance=Visualization.FlightGear.generateRunScript.offsetDistance  OffsetAzimuth=Visualization.FlightGear.generateRunScript.offsetAzimuth  InstallScenery=off  DisableShaders=off  OriginAddress=127.0.0.1  DestinationPort=Visualization.FlightGear.generateRunScript.destinationPort  OriginPort=5505  LocalAddress=127.0.0.1  OutputFileName=runfg.bat  FlightGearBaseDirectory=C:\Program Files\FlightGear
  Mux : Mux  Inputs=2
  Terminator : Terminator
  wires:
  States/1 -> Bus Selector/1
  Bus Selector/1 -> Mux/1  "<LLA>"
  Bus Selector/2 -> Mux/2  "<Euler>"
  Mux/1 -> FlightGear Preconfigured 6DoF Animation/1
  Commands/1 -> Terminator/1

== system flightSimulation/Visualization/Visualization/Scopes ==
  Commands : Inport
  States : Inport  Port=2
  Bus Creator : BusCreator  Inputs=2
  Bus Selector : BusSelector  OutputSignals=States.V_body,States.Euler,States.X_ned
  Euler : Scope
  V_body : Scope
  X_ned : Scope
  wires:
  Commands/1 -> Bus Creator/1  "Commands"
  States/1 -> Bus Creator/2  "States"
  Bus Creator/1 -> Bus Selector/1
  Bus Selector/1 -> V_body/1  "<V_body>"
  Bus Selector/2 -> Euler/1  "<Euler>"
  Bus Selector/3 -> X_ned/1  "<X_ned>"

== system flightSimulation/Visualization/Visualization/Simulink 3D ==
  Commands : Inport
  States : Inport  Port=2
  Axes to VR Axes : Subsystem
  Bus Selector : BusSelector  OutputSignals=Euler,X_ned
  Euler to VR : Subsystem
  Rate Transition : RateTransition
  Rate Transition1 : RateTransition
  Terminator : Terminator
  VR Sink : vrlib/VR Sink  InstantiateOnLoad=on  SampleTime=40*Ts  ViewEnable=on  RemoteChange=off  RemoteView=off  FieldsWritten=QuadBody.rotation.4.1.1.double#QuadBody.translation.3.1.1.double  WorldFileName=asbFlightSimulationWorld.wrl  AutoView=on  VideoDimensions=[]  AllowVariableSize=off
      settings: SourceProductBaseCode=VR
  wires:
  Commands/1 -> Terminator/1
  States/1 -> Bus Selector/1
  Euler to VR/1(Axis Angle) -> Rate Transition/1
  Axes to VR Axes/1(Xe VR) -> Rate Transition1/1
  Bus Selector/1 -> Euler to VR/1(Euler Angles)  "<Euler>"
  Bus Selector/2 -> Axes to VR Axes/1(Xe)  "<X_ned>"
  Rate Transition/1 -> VR Sink/1
  Rate Transition1/1 -> VR Sink/2

== system flightSimulation/Visualization/Visualization/Workspace ==
  Commands : Inport
  States : Inport  Port=2
  Bus Selector : BusSelector  OutputSignals=V_body,Omega_body,Euler
  Bus Selector1 : BusSelector  OutputSignals=roll_cmd,pitch_cmd,yaw_cmd,throttle_cmd
  CommandsOut : ToWorkspace  VariableName=CommandsOut  SaveFormat=Timeseries  SampleTime=0.01
  Mux : Mux  Inputs=3
  Mux1 : Mux
  StatesOut : ToWorkspace  VariableName=statesOut  SaveFormat=Timeseries  SampleTime=0.01
  wires:
  States/1 -> Bus Selector/1
  Bus Selector/2 -> Mux/2  "<Omega_body>"
  Bus Selector/3 -> Mux/3  "<Euler>"
  Bus Selector/1 -> Mux/1  "<V_body>"
  Commands/1 -> Bus Selector1/1
  Bus Selector1/2 -> Mux1/2  "<pitch_cmd>"
  Bus Selector1/1 -> Mux1/1  "<roll_cmd>"
  Bus Selector1/4 -> Mux1/4  "<throttle_cmd>"
  Bus Selector1/3 -> Mux1/3  "<yaw_cmd>"
  Mux1/1 -> CommandsOut/1
  Mux/1 -> StatesOut/1

== system flightSimulation/Nonlinear/Plant/Subsystem/Subsystem1 ==
  F : Inport
  g_ned : Inport  Port=2
  Rn2b : Inport  Port=3
  Add : Sum
  Gain : Gain  Gain=mass
  Product : Product  Multiplication=Matrix(*)
  F_b : Outport
  wires:
  g_ned/1 -> Gain/1
  Rn2b/1 -> Product/1
  Gain/1 -> Product/2
  Product/1 -> Add/1  "G_b"
  F/1 -> Add/2
  Add/1 -> F_b/1

== system flightSimulation/Subsystem/ADRC_allocator/Subsystem2/Signal Builder ==
  Demux : Demux  Tag=STV Demux
  FromWs : FromWorkspace  Tag=STV FromWs  VariableName=tuvar  SampleTime=0
      SigBuilderData=|
      | common.afterFinalStr = 'Extrapolate'
      | common.sampleTime = 0
      | dataSet.timeRange = [0 100]
      | dataSet.name = 'Group 1'
      | sbobj.Groups.Name = 'Group 1'
      | sbobj.Groups.Signals(1).Name = 'roll_cmd'
      | sbobj.Groups.Signals(1).XData = [0 0.5 5 100]
      | sbobj.Groups.Signals(1).YData = [0 0 -0.157079632679 -0.157079632679]
      | sbobj.Groups.Signals(2).Name = 'picth_cmd'
      | sbobj.Groups.Signals(2).XData = [0 30 30 100]
      | sbobj.Groups.Signals(2).YData = [-0.0045 -0.0045 0.3 0.3]
      | sbobj.Groups.Signals(3).Name = 'yaw_cmd'
      | sbobj.Groups.Signals(3).XData = [0 30 30 100]
      | sbobj.Groups.Signals(3).YData = [0.0779 0.0779 0.2 0.2]
      | sbobj.Groups.Signals(4).Name = 'throttle_cmd'
      | sbobj.Groups.Signals(4).XData = [0 0.55 5 100]
      | sbobj.Groups.Signals(4).YData = [0 0 -0.17 -0.17]
      | sbobj.Groups.TimeRange = [0 100]
  roll_cmd : Outport  Tag=STV Outport
  picth_cmd : Outport  Tag=STV Outport  Port=2
  yaw_cmd : Outport  Tag=STV Outport  Port=3
  throttle_cmd : Outport  Tag=STV Outport  Port=4
  wires:
  Demux/1 -> roll_cmd/1
  FromWs/1 -> Demux/1
  Demux/2 -> picth_cmd/1
  Demux/3 -> yaw_cmd/1
  Demux/4 -> throttle_cmd/1

== system flightSimulation/Subsystem/ADRC_allocator1/Subsystem2/Signal Builder ==
  Demux : Demux  Tag=STV Demux
  FromWs : FromWorkspace  Tag=STV FromWs  VariableName=tuvar  SampleTime=0
      SigBuilderData=|
      | common.afterFinalStr = 'Extrapolate'
      | common.sampleTime = 0
      | dataSet.timeRange = [0 100]
      | dataSet.name = 'Group 1'
      | sbobj.Groups.Name = 'Group 1'
      | sbobj.Groups.Signals(1).Name = 'roll_cmd'
      | sbobj.Groups.Signals(1).XData = [0 0.5 8 100]
      | sbobj.Groups.Signals(1).YData = [0 0 -0.13962634016 -0.13962634016]
      | sbobj.Groups.Signals(2).Name = 'picth_cmd'
      | sbobj.Groups.Signals(2).XData = [0 30 100]
      | sbobj.Groups.Signals(2).YData = [0 0 0]
      | sbobj.Groups.Signals(3).Name = 'yaw_cmd'
      | sbobj.Groups.Signals(3).XData = [0 30 30 100]
      | sbobj.Groups.Signals(3).YData = [0.0779 0.0779 0.2 0.2]
      | sbobj.Groups.Signals(4).Name = 'throttle_cmd'
      | sbobj.Groups.Signals(4).XData = [0 0.55 5 100]
      | sbobj.Groups.Signals(4).YData = [0 0 -0.17 -0.17]
      | sbobj.Groups.TimeRange = [0 100]
  roll_cmd : Outport  Tag=STV Outport
  picth_cmd : Outport  Tag=STV Outport  Port=2
  yaw_cmd : Outport  Tag=STV Outport  Port=3
  throttle_cmd : Outport  Tag=STV Outport  Port=4
  wires:
  Demux/1 -> roll_cmd/1
  FromWs/1 -> Demux/1
  Demux/2 -> picth_cmd/1
  Demux/3 -> yaw_cmd/1
  Demux/4 -> throttle_cmd/1

== system flightSimulation/Subsystem/ADRC_allocator1/Subsystem2/actuator model ==
  cmd_c : Inport
  Demux3 : Demux
  Mux1 : Mux
  Transfer Fcnnon{1..4} (4 alike) : TransferFcn  Numerator=45  Denominator=[1 45]
  Out1 : Outport
  wires:
  Demux3/1 -> Transfer Fcnnon4/1
  Transfer Fcnnon3/1 -> Mux1/4  "c4"
  Demux3/2 -> Transfer Fcnnon1/1
  Demux3/3 -> Transfer Fcnnon2/1
  Transfer Fcnnon4/1 -> Mux1/1  "c1"
  Demux3/4 -> Transfer Fcnnon3/1
  Mux1/1 -> Out1/1
  Transfer Fcnnon2/1 -> Mux1/3  "c3"
  Transfer Fcnnon1/1 -> Mux1/2  "c2"
  cmd_c/1 -> Demux3/1

== system flightSimulation/Subsystem/ADRC_allocator1/Subsystem2/control allocation ==
  note: 1) Add Subsystem or Model blocks as valid variant choices.
      | 2) You cannot connect blocks at this level. At simulation, connectivity is automatically
      | determined, based on the active variant and port name matching.
  u : Inport
  d : Inport  Port=2
  c : Inport  Port=3
  dir : Subsystem  VariantControl=allocatiom_method==1
  inv : Subsystem  VariantControl=allocatiom_method==0
  pro : Subsystem  VariantControl=allocatiom_method==2
  qp : Subsystem  VariantControl=allocatiom_method==3
  Out1 : Outport

== system flightSimulation/Subsystem/ADRC_allocator1/Subsystem2/noise1 ==
  In1 : Inport
  Analog Filter Design{,1..3} (4 alike) : dsparch4/Analog Filter Design  method=Butterworth  filttype=Lowpass  N=1  Wlo=50  Whi=80  Rp=2  Rs=40
  Colored Noise1 : dspsrcs4/Colored Noise  Color=pink  InverseFrequencyPower=2  NumChannels=1  OutputDataType=double  SamplesPerFrame=1  SampleTime=0.005  RandomStream=mt19937ar with seed  Seed=randperm(100000,1)  SimulateUsing=Interpreted execution
      settings: SourceProductName=DSP System Toolbox  SourceProductBaseCode=DS
  Colored Noise2 : dspsrcs4/Colored Noise  Color=blue  InverseFrequencyPower=2  NumChannels=1  OutputDataType=double  SamplesPerFrame=1  SampleTime=0.005  RandomStream=mt19937ar with seed  Seed=randperm(100000,1)  SimulateUsing=Interpreted execution
      settings: SourceProductName=DSP System Toolbox  SourceProductBaseCode=DS
  Colored Noise3 : dspsrcs4/Colored Noise  Color=pink  InverseFrequencyPower=2  NumChannels=1  OutputDataType=double  SamplesPerFrame=1  SampleTime=0.01  RandomStream=mt19937ar with seed  Seed=randperm(100000,1)  SimulateUsing=Interpreted execution
      settings: SourceProductName=DSP System Toolbox  SourceProductBaseCode=DS
  Colored Noise5 : dspsrcs4/Colored Noise  Color=pink  InverseFrequencyPower=2  NumChannels=1  OutputDataType=double  SamplesPerFrame=1  SampleTime=0.01  RandomStream=mt19937ar with seed  Seed=randperm(100000,1)  SimulateUsing=Interpreted execution
      settings: SourceProductName=DSP System Toolbox  SourceProductBaseCode=DS
  Demux : Demux
  Gain{1..4} (4 alike) : Gain  Gain=0.001
  Mux : Mux
  Random Number : RandomNumber  Variance=8.1663e-6  Seed=randperm(100000,1)
  Random Number1 : RandomNumber  Variance=3.5671e-6  Seed=randperm(100000,1)
  Random Number2 : RandomNumber  Variance=7.1339e-6  Seed=randperm(100000,1)
  Random Number3 : RandomNumber  Variance=5.2533e-6  Seed=randperm(100000,1)
  Scope{,1..3} (4 alike) : Scope  NumInputPorts=2
  Sum{1..4} (4 alike) : Sum  Inputs=|++
  Out1 : Outport
  wires:
  Sum4/1 -> Mux/3, Scope2/2, Analog Filter Design2/1
  Sum3/1 -> Mux/2, Analog Filter Design1/1, Scope1/2
  Sum1/1 -> Mux/1, Analog Filter Design/1, Scope/2
  In1/1 -> Demux/1
  Mux/1 -> Out1/1
  Demux/4 -> Sum2/2
  Sum2/1 -> Mux/4, Analog Filter Design3/1, Scope3/2
  Demux/1 -> Sum1/2
  Demux/2 -> Sum3/2
  Demux/3 -> Sum4/2
  Colored Noise2/1 -> Gain2/1
  Gain2/1 -> Sum4/1, Sum1/1
  Colored Noise1/1 -> Gain1/1
  Colored Noise3/1 -> Gain3/1
  Colored Noise5/1 -> Gain4/1
  Gain1/1 -> Sum2/1, Sum3/1
  Analog Filter Design/1 -> Scope/1
  Analog Filter Design1/1 -> Scope1/1
  Analog Filter Design2/1 -> Scope2/1
  Analog Filter Design3/1 -> Scope3/1

== system flightSimulation/Subsystem/PID_allocator/Subsystem2/Signal Builder ==
  Demux : Demux  Tag=STV Demux
  FromWs : FromWorkspace  Tag=STV FromWs  VariableName=tuvar  SampleTime=0
      SigBuilderData=|
      | common.afterFinalStr = 'Extrapolate'
      | common.sampleTime = 0
      | dataSet.timeRange = [0 100]
      | dataSet.name = 'Group 1'
      | sbobj.Groups.Name = 'Group 1'
      | sbobj.Groups.Signals(1).Name = 'roll_cmd'
      | sbobj.Groups.Signals(1).XData = [0 4 10 10 100]
      | sbobj.Groups.Signals(1).YData = [0.0045 0 -0.0872665 -0.0872664625997 -0.0872664625997]
      | sbobj.Groups.Signals(2).Name = 'picth_cmd'
      | sbobj.Groups.Signals(2).XData = [0 30 30 100]
      | sbobj.Groups.Signals(2).YData = [-0.0045 -0.0045 0.3 0.3]
      | sbobj.Groups.Signals(3).Name = 'yaw_cmd'
      | sbobj.Groups.Signals(3).XData = [0 30 30 100]
      | sbobj.Groups.Signals(3).YData = [0.0779 0.0779 0.2 0.2]
      | sbobj.Groups.Signals(4).Name = 'throttle_cmd'
      | sbobj.Groups.Signals(4).XData = [0 100]
      | sbobj.Groups.Signals(4).YData = [0 0]
      | sbobj.Groups.TimeRange = [0 100]
  roll_cmd : Outport  Tag=STV Outport
  picth_cmd : Outport  Tag=STV Outport  Port=2
  yaw_cmd : Outport  Tag=STV Outport  Port=3
  throttle_cmd : Outport  Tag=STV Outport  Port=4
  wires:
  Demux/1 -> roll_cmd/1
  FromWs/1 -> Demux/1
  Demux/2 -> picth_cmd/1
  Demux/3 -> yaw_cmd/1
  Demux/4 -> throttle_cmd/1

== system flightSimulation/Subsystem/PID_allocator1/Subsystem2/Signal Builder ==
  Demux : Demux  Tag=STV Demux
  FromWs : FromWorkspace  Tag=STV FromWs  VariableName=tuvar  SampleTime=0
      SigBuilderData=|
      | common.afterFinalStr = 'Extrapolate'
      | common.sampleTime = 0
      | dataSet.timeRange = [0 100]
      | dataSet.name = 'Group 1'
      | sbobj.Groups.Name = 'Group 1'
      | sbobj.Groups.Signals(1).Name = 'roll_cmd'
      | sbobj.Groups.Signals(1).XData = [0 4 10 10 100]
      | sbobj.Groups.Signals(1).YData = [0.0045 0 -0.0872665 -0.0872664625997 -0.0872664625997]
      | sbobj.Groups.Signals(2).Name = 'picth_cmd'
      | sbobj.Groups.Signals(2).XData = [0 30 30 100]
      | sbobj.Groups.Signals(2).YData = [-0.0045 -0.0045 0.3 0.3]
      | sbobj.Groups.Signals(3).Name = 'yaw_cmd'
      | sbobj.Groups.Signals(3).XData = [0 30 30 100]
      | sbobj.Groups.Signals(3).YData = [0.0779 0.0779 0.2 0.2]
      | sbobj.Groups.Signals(4).Name = 'throttle_cmd'
      | sbobj.Groups.Signals(4).XData = [0 100]
      | sbobj.Groups.Signals(4).YData = [0 0]
      | sbobj.Groups.TimeRange = [0 100]
  roll_cmd : Outport  Tag=STV Outport
  picth_cmd : Outport  Tag=STV Outport  Port=2
  yaw_cmd : Outport  Tag=STV Outport  Port=3
  throttle_cmd : Outport  Tag=STV Outport  Port=4
  wires:
  Demux/1 -> roll_cmd/1
  FromWs/1 -> Demux/1
  Demux/2 -> picth_cmd/1
  Demux/3 -> yaw_cmd/1
  Demux/4 -> throttle_cmd/1

== system flightSimulation/Visualization/Visualization/Simulink 3D/Axes to VR Axes ==
  Xe : Inport
  Demux : Demux  Outputs=3
  Mux : Mux  Inputs=3
  rad-->deg1 : Gain  Gain=-1  SaturateOnIntegerOverflow=on  OutDataTypeStr=Inherit: Same as input  ParamDataTypeStr=Inherit: Same as input
  Xe VR : Outport
  wires:
  Xe/1 -> Demux/1
  Demux/1 -> Mux/1
  Demux/3 -> rad-->deg1/1
  Mux/1 -> Xe VR/1
  rad-->deg1/1 -> Mux/2
  Demux/2 -> Mux/3

== system flightSimulation/Visualization/Visualization/Simulink 3D/Euler to VR ==
  Euler Angles : Inport
  Axis Angle Vector : Subsystem
  Mux : Mux  Inputs=2
  Mux1 : Mux  Inputs=2
  Mux2 : Mux  Inputs=2
  Quaternion Multiplication (Pitch & Yaw) : aerolibutil/Quaternion Multiplication
  Quaternion Multiplication (Roll) : aerolibutil/Quaternion Multiplication
  Quaternion Normalization : Subsystem
  Quaternion Normalization1 : Subsystem
  Quaternion Normalization2 : Subsystem
  Selector : Selector  InputPortWidth=3  IndexOptions=Index vector (dialog)  Indices=[3]  OutputSizes=1
  Selector1 : Selector  InputPortWidth=3  IndexOptions=Index vector (dialog)  Indices=[2]  OutputSizes=1
  Selector2 : Selector  InputPortWidth=3  IndexOptions=Index vector (dialog)  Indices=[1]  OutputSizes=1
  Vr Pitch Axes : Constant  Value=[0 0 1]
  Vr Roll Axes : Constant  Value=[1 0 0]
  Vr Yaw Axes : Constant  Value=[0 -1 0]
  Axis Angle : Outport
  wires:
  Quaternion Multiplication (Roll)/1 -> Axis Angle Vector/1(e0)
  Axis Angle Vector/1(e0_norm) -> Axis Angle/1
  Quaternion Normalization/1(e0_norm) -> Quaternion Multiplication (Roll)/2
  Quaternion Normalization2/1(e0_norm) -> Quaternion Multiplication (Pitch & Yaw)/1
  Quaternion Normalization1/1(e0_norm) -> Quaternion Multiplication (Pitch & Yaw)/2
  Mux2/1 -> Quaternion Normalization2/1(e0)
  Mux1/1 -> Quaternion Normalization1/1(e0)
  Mux/1 -> Quaternion Normalization/1(e0)
  Selector/1 -> Mux2/1
  Vr Yaw Axes/1 -> Mux2/2
  Selector1/1 -> Mux1/1
  Vr Pitch Axes/1 -> Mux1/2
  Selector2/1 -> Mux/1
  Vr Roll Axes/1 -> Mux/2
  Euler Angles/1 -> Selector2/1, Selector1/1, Selector/1
  Quaternion Multiplication (Pitch & Yaw)/1 -> Quaternion Multiplication (Roll)/1

== system flightSimulation/Subsystem/ADRC_allocator1/Subsystem2/control allocation/dir ==
  u : Inport
  d : Inport  Port=2
  c : Inport  Port=3
  Mux : Mux  Inputs=2
  S-Function2 : S-Function  FunctionName=s_dir  SFunctionDeploymentMode=off  EnableBusSupport=off
  Sum : Sum  Inputs=|+-
  Out1 : Outport
  wires:
  S-Function2/1 -> Out1/1
  u/1 -> Sum/1
  Sum/1 -> Mux/1
  d/1 -> Sum/2
  Mux/1 -> S-Function2/1
  c/1 -> Mux/2

== system flightSimulation/Subsystem/ADRC_allocator1/Subsystem2/control allocation/inv ==
  u : Inport
  d : Inport  Port=2
  Sum : Sum  Inputs=|+-
  inv : MATLAB Function  TreatAsAtomicUnit=on
  Out1 : Outport
  wires:
  inv/1(y) -> Out1/1
  u/1 -> Sum/1
  Sum/1 -> inv/1(u)
  d/1 -> Sum/2

== system flightSimulation/Subsystem/ADRC_allocator1/Subsystem2/control allocation/pro ==
  u : Inport
  d : Inport  Port=2
  c : Inport  Port=3
  Mux : Mux  Inputs=3
  S-Function1 : S-Function  FunctionName=s_prio1  SFunctionDeploymentMode=off  EnableBusSupport=off
  Out1 : Outport
  wires:
  Mux/1 -> S-Function1/1
  S-Function1/1 -> Out1/1
  u/1 -> Mux/1
  d/1 -> Mux/2
  c/1 -> Mux/3

== system flightSimulation/Subsystem/ADRC_allocator1/Subsystem2/control allocation/qp ==
  u : Inport
  d : Inport  Port=2
  QP control allocator : qcatlib/QP control allocator  B=B  plim=[umin umax]  rlim=[]  T=0.01  Wv=eye(3)  Wu=eye(4)  ud=zeros(4,1)  alg=WLS  imax=100  gam=1e4  tol=1e-4
      settings: SourceProductName=QP Control Allocation Toolbox
  Sum : Sum  Inputs=|+-
  Out1 : Outport
  wires:
  u/1 -> Sum/1
  QP control allocator/1 -> Out1/1
  d/1 -> Sum/2
  Sum/1 -> QP control allocator/1

== system flightSimulation/Visualization/Visualization/Simulink 3D/Euler to VR/Axis Angle Vector ==
  e0 : Inport
  2 : Gain  Gain=2  SaturateOnIntegerOverflow=on  OutDataTypeStr=Inherit: Same as input  ParamDataTypeStr=Inherit: Same as input
  Constant : Constant  Value=1e-6
  Demux : Demux  Outputs=[1 3 ]
  Mux : Mux  Inputs=2
  Product : Product  Inputs=*/  SaturateOnIntegerOverflow=on  InputSameDT=on  OutDataTypeStr=Inherit: Same as first input
  Switch : Switch  Criteria=u2 ~= 0
  Trigonometric Function : Trigonometry
  Trigonometric Function2 : Trigonometry  Operator=acos
  e0_norm : Outport
  wires:
  Demux/1 -> Trigonometric Function2/1
  Demux/2 -> Product/1
  Mux/1 -> e0_norm/1
  Product/1 -> Mux/1
  2/1 -> Mux/2
  Trigonometric Function/1 -> Switch/1, Switch/2
  Trigonometric Function2/1 -> Trigonometric Function/1, 2/1
  e0/1 -> Demux/1
  Constant/1 -> Switch/3
  Switch/1 -> Product/2

== system flightSimulation/Visualization/Visualization/Simulink 3D/Euler to VR/Quaternion Normalization ==
  e0 : Inport
  1/2 : Gain  Gain=1/2  SaturateOnIntegerOverflow=on  OutDataTypeStr=Inherit: Same as input  ParamDataTypeStr=Inherit: Same as input
  Demux : Demux  Outputs=[1 3]
  Mux : Mux  Inputs=2
  Product : Product  SaturateOnIntegerOverflow=on  InputSameDT=on  OutDataTypeStr=Inherit: Same as first input
  Trigonometric Function : Trigonometry
  Trigonometric Function1 : Trigonometry  Operator=cos
  e0_norm : Outport
  wires:
  Trigonometric Function1/1 -> Mux/1
  Demux/2 -> Product/2
  Demux/1 -> 1/2/1
  Mux/1 -> e0_norm/1
  Product/1 -> Mux/2
  Trigonometric Function/1 -> Product/1
  1/2/1 -> Trigonometric Function1/1, Trigonometric Function/1
  e0/1 -> Demux/1

== system flightSimulation/Visualization/Visualization/Simulink 3D/Euler to VR/Quaternion Normalization1 ==
  e0 : Inport
  1/2 : Gain  Gain=1/2  SaturateOnIntegerOverflow=on  OutDataTypeStr=Inherit: Same as input  ParamDataTypeStr=Inherit: Same as input
  Demux : Demux  Outputs=[1 3]
  Mux : Mux  Inputs=2
  Product : Product  SaturateOnIntegerOverflow=on  InputSameDT=on  OutDataTypeStr=Inherit: Same as first input
  Trigonometric Function : Trigonometry
  Trigonometric Function1 : Trigonometry  Operator=cos
  e0_norm : Outport
  wires:
  e0/1 -> Demux/1
  1/2/1 -> Trigonometric Function/1, Trigonometric Function1/1
  Trigonometric Function/1 -> Product/1
  Product/1 -> Mux/2
  Mux/1 -> e0_norm/1
  Demux/1 -> 1/2/1
  Demux/2 -> Product/2
  Trigonometric Function1/1 -> Mux/1

== system flightSimulation/Visualization/Visualization/Simulink 3D/Euler to VR/Quaternion Normalization2 ==
  e0 : Inport
  1/2 : Gain  Gain=1/2  SaturateOnIntegerOverflow=on  OutDataTypeStr=Inherit: Same as input  ParamDataTypeStr=Inherit: Same as input
  Demux : Demux  Outputs=[1 3]
  Mux : Mux  Inputs=2
  Product : Product  SaturateOnIntegerOverflow=on  InputSameDT=on  OutDataTypeStr=Inherit: Same as first input
  Trigonometric Function : Trigonometry
  Trigonometric Function1 : Trigonometry  Operator=cos
  e0_norm : Outport
  wires:
  Trigonometric Function1/1 -> Mux/1
  Demux/2 -> Product/2
  Demux/1 -> 1/2/1
  Mux/1 -> e0_norm/1
  Product/1 -> Mux/2
  Trigonometric Function/1 -> Product/1
  1/2/1 -> Trigonometric Function1/1, Trigonometric Function/1
  e0/1 -> Demux/1

== matlab function flightSimulation/Subsystem/PID_allocator/舵机偏角输入eso/MATLAB Function2 ==
  data: u input; y output
function y = fcn(u)
U1=u(1);
U2=u(2);
U3=u(3);
A=0.3491;

D=[-1  0  1;
    0 -1  1;
    1  0  1;
    0  1  1];
% D
D_=1*[-0.5000         0              0.5000         0;
         0           -0.5000         0              0.5000;
       0.2500         0.2500         0.2500         0.2500];
% pinv(D)
kc1=2.7;% 2.8
kc2=3.2;% 3.3
l_1=0.17078793;
l_2=0.06647954;
K=1*[-kc1*l_1    0        kc1*l_1     0;
      0      -kc1*l_1     0        kc1*l_1;
      kc2*l_2   kc2*l_2    kc2*l_2    kc2*l_2];
K_=pinv(K);
I_x=0.025483;
I_y=0.025504;
I_z=0.00562;
I=[I_x 0 0;0 I_y 0;0 0 I_z];
a=A-abs(U1);
b=A-abs(U2);
D_s=[-1  0 (2*a)/(a+b);
      0 -1  (2*b)/(a+b);
      1  0  (2*a)/(a+b);
      0  1 (2*b)/(a+b)];
    D=[-1  0  1;
      0 -1  1;
      1  0  1;
      0  1  1];
y=zeros(3,1);
y=I\(K*D)*([U1;U2;U3]);% K*D=K*D_s
% I\(K*D)*([U1;U2;U3])=扰动加速度

== matlab function flightSimulation/Subsystem/PID/舵面分配/inv ==
  data: u input; y output
function y = fcn(u)
U = [u(1);u(2);u(3)];
% M=crossover_point([0;0;0],e);
% if (norm(e)>norm(M))
%     U=M;
% else
%     U=e;
% end 
% B=[-0.5   0       0.5   0;
%     0  -0.5    0       0.5;
%     0.25   0.25   0.25   0.25];
kc1=3.157;% 2.8
kc2=3.157;% 3.3
l_1=0.17078793;
l_2=0.06647954;
B=1*[-kc1*l_1    0        kc1*l_1     0;
      0      -kc1*l_1     0        kc1*l_1;
      kc2*l_2   kc2*l_2    kc2*l_2    kc2*l_2]; 
% u(1)=Constrain(u(1),umin(1),umax(1));
% u(2)=Constrain(u(2),umin(2),umax(2));
% u(3)=Constrain(u(3),umin(3),umax(3));
% u(4)=Constrain(u(4),umin(4),umax(4));
c=pinv(B)*U;
y=[c(1);c(2);c(3);c(4)];

== matlab function flightSimulation/Subsystem/PID_allocator/MATLAB Function ==
  data: u input; y output
function y = Eulerrate2pqr(u)
Roll=u(4);
Pitch=u(5);
Q=[1    sin(Roll)*tan(Pitch)    cos(Roll)*tan(Pitch);
   0        cos(Roll)               -sin(Roll);
   0    sin(Roll)*sec(Pitch)    cos(Roll)*sec(Pitch)];
y = Q\[u(1);u(2);u(3)];

== matlab function flightSimulation/Subsystem/PID_allocator/MATLAB Function1 ==
  data: u input; y output
function y = Yawcontrol(u)
if u<-pi
    a=u+2*pi;
elseif u>=pi
    a=u-2*pi;
else   
    a=u;
end
y = a;

== matlab function flightSimulation/Subsystem/PID_allocator1/MATLAB Function ==
  data: u input; y output
function y = Eulerrate2pqr(u)
Roll=u(4);
Pitch=u(5);
Q=[1    sin(Roll)*tan(Pitch)    cos(Roll)*tan(Pitch);
   0        cos(Roll)               -sin(Roll);
   0    sin(Roll)*sec(Pitch)    cos(Roll)*sec(Pitch)];
y = Q\[u(1);u(2);u(3)];

== matlab function flightSimulation/Subsystem/PID_allocator/Subsystem2/inv ==
  data: u input; y output
function y = fcn(u)
U = [u(1);u(2);u(3)];
% M=crossover_point([0;0;0],e);
% if (norm(e)>norm(M))
%     U=M;
% else
%     U=e;
% end 
% B=[-0.5   0       0.5   0;
%     0  -0.5    0       0.5;
%     0.25   0.25   0.25   0.25];
kc1=3.157;% 2.8
kc2=3.157;% 3.3
l_1=0.17078793;
l_2=0.06647954;
B=1*[-kc1*l_1    0        kc1*l_1     0;
      0      -kc1*l_1     0        kc1*l_1;
      kc2*l_2   kc2*l_2    kc2*l_2    kc2*l_2];  
% u(1)=Constrain(u(1),umin(1),umax(1));
% u(2)=Constrain(u(2),umin(2),umax(2));
% u(3)=Constrain(u(3),umin(3),umax(3));
% u(4)=Constrain(u(4),umin(4),umax(4));
c=pinv(B)*U;
y=[c(1);c(2);c(3);c(4)];

== matlab function flightSimulation/Subsystem/PID_allocator1/MATLAB Function1 ==
  data: u input; y output
function y = Yawcontrol(u)
if u<-pi
    a=u+2*pi;
elseif u>=pi
    a=u-2*pi;
else   
    a=u;
end
y = a;
